simulink model "ls_estimator"  (R2024b)
settings: Solver=VariableStepAuto  StartTime=0.0  StopTime=10.0  RelTol=1e-3
settings Model: Creator=djd14  LastModifiedBy=djd14

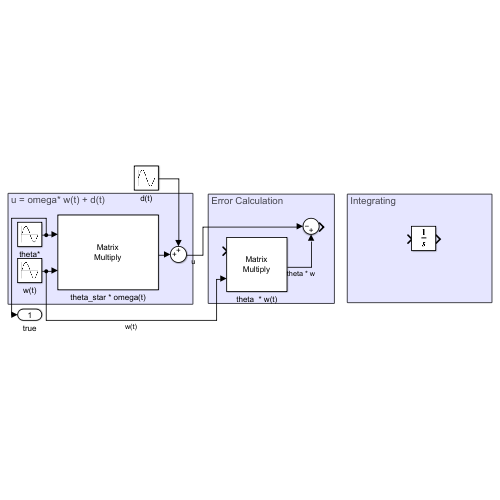
[thumbnail: Simulink's stored preview of the top-level diagram]
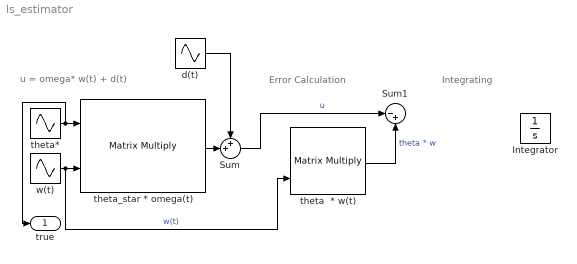
== system ls_estimator ==
  note: Integrating
  note: u = omega* w(t) + d(t)
  note: Error Calculation
  Integrator : Integrator
  Sum : Sum  Inputs=++|
  Sum1 : Sum  Inputs=|-+
  d(t) : Sin  Amplitude=0  Frequency=20  SampleTime=0
  theta  * w(t) : Product  Multiplication=Matrix(*)
  theta* : Sin  Amplitude=0.5  Bias=1  Frequency=0.5  SampleTime=0
  theta_star * omega(t) : Product  Multiplication=Matrix(*)
  w(t) : Sin  SampleTime=0
  true : Outport
  wires:
  theta*/1 -> true/1, theta_star * omega(t)/1
  d(t)/1 -> Sum/1
  Sum/1 -> Sum1/1  "u"
  w(t)/1 -> theta  * w(t)/2, theta_star * omega(t)/2  "w(t)"
  theta  * w(t)/1 -> Sum1/2  "theta * w"
  theta_star * omega(t)/1 -> Sum/2
